simulink model "CDD_ISP_beautified"  (R2022b)
settings: Solver=ode1  StartTime=0.0  StopTime=0.2  FixedStep=ctrlConst.TsSwitch  MaxStep=1e-6  RelTol=1e-3  EnableMultiTasking=on
undefined symbols (not defined in the file): agNegTrans_C, ECM, f32_P_AngleCompCur, f32_P_AngleCompVol, f32_SpeedFltCoef, facAdc2iPh_C, facAdc2uDclnk_C, g_msgCore0to2_depth, g_msgCore0to2_detlaAngle_single, g_msgCore0to2_fbw, g_msgCore0to2_L1, g_msgCore0to2_L2, g_msgCore0to2_N111, g_msgCore0to2_N222, g_msgCore0to2_pwmFrqSet, g_msgCore0to2_wb, IdROL_C, iPhaMax_C, iPhaMin_C, offsAgRtrElec_C, rotatedirection_C, SC_p_P, SC_pRsv_P, tauUdcPT1_C, Ts_10ms, Tsw, uDcMax_C, uDcMin_C
libraries: MathLib x6, simulink x4
(part 2 of 2)

== matlab function CDD_ISP_beautified/ISP_ResolverSel/MATLAB Function ==
  data: x0 input; y output; x1 input; x2 input; y1 input; y2 input; wc input; wb input
function y = fcn(x0,x1,x2,y1,y2,wc,wb)


persistent reset;
%ISC_agOffs_P = int16(Angleoffset_Init);  %
if isempty(reset)
    reset = boolean(1);
    a0=single(0);
    a1=single(0);
    y1=single(0);
    y2=single(0);
end



Ts= single(1/16000);
a0= single(4+wc^2*Ts^2);
a1= single(2*Ts^2*wc^2-8);
a2= single(a0);
b0 =single(4+wc^2*Ts^2+2*wb*Ts);
b1 =single(a1);
b2 =single(4+wc^2*Ts^2-2*wb*Ts);

temp = single(a0*x0+a1*x1+a2*x2-b1*y1-b2*y2);


if(wc == single(0))
temp = x0;
end
% if(n_abs<=500)
% 
% y=x0;
% 
% else
y= single(temp);

%end

== matlab function CDD_ISP_beautified/CddPhaCur&CddRslvr/CddRslvr_CalnPosCaln/MATLAB Function ==
  data: omega_hat_K_1 output; omega_hat_K input; theta_hat_K_1 output; theta_meas_k input; theta_hat_k input; L1 input; L2 input
function [omega_hat_K_1,theta_hat_K_1]    = fcn(omega_hat_K,theta_meas_k,theta_hat_k,L1,L2)

persistent reset;
if isempty(reset)
    reset = boolean(1);
%     theta_hat_K_1 = single(0);
%     omega_hat_K_1 = sinle(0);
    omega_hat_K =  single(0);
    theta_hat_k = single(0);
end
Ts= single(1/16000);
ek = theta_meas_k - theta_hat_k;
theta_hat_K_1 = theta_hat_k + (omega_hat_K + L1 * ek)* Ts;
omega_hat_K_1 = omega_hat_K + L2 * ek * Ts;



% # 输入：theta_meas(k) = 编码器实测机械位置(rad)
% # 输出：omega_hat(k) = 平滑转速(rad/s)
% # 调参：l1, l2（观测器增益），dt = 控制周期(s)
% 
% # 1. 计算位置误差（核心修正项）
% e(k) = theta_meas(k) - theta_hat(k)
% 
% # 2. 更新内部预测位置（仅用于误差计算，不输出）
% theta_hat(k+1) = theta_hat(k) + [omega_hat(k) + l1 * e(k)] * dt
% 
% # 3. 更新输出转速（无参数，仅用误差修正）
% omega_hat(k+1) = omega_hat(k) + l2 * e(k) * dt
